simulink model "topology2_module"  (R2013a)
settings: Solver=ode4  StartTime=0.0  StopTime=0.02  FixedStep=Ts  RelTol=1e-3
values from neighbouring files (symbols this model uses):
  enable = zeros(1,max_number_module)    [immd_base_varyingmod.m]
  Lload = Xload/wout_fund    [acemp_sixth.m]    (also in immd_base_varyingmod.m = Xload/wout; immd_design_elen.m = Xload/wout; immd_efficiency.m = Xload/wout; immd_simulation_base.m)
  ma = 1    [IMMD_design_tool_v01.m]    (also in IMMD_design_tool_v02.m = 0.9; immd_base_varyingmod.m; immd_design_elen.m = 0.8; immd_efficiency.m = 0.85)
  phase = zeros(1,max_number_module)    [immd_base_varyingmod.m]    (also in immd_design_elen.m = [0 0 0 0]; immd_simulation_base.m = zeros(1,n))
  Rload = Zload*pf    [acemp_sixth.m]    (also in immd_base_varyingmod.m; immd_design_elen.m; immd_efficiency.m; immd_simulation_base.m)
  Ts = 1e-6    (= 1e-06)    [acemp_sixth.m]    (also in immd_base_varyingmod.m = 1e-05; immd_design_elen.m; immd_efficiency.m; immd_simulation_base.m)
  Vdc = (3/pi)*Vs_ll*sqrt(2)    [IMMD_design_tool_v01.m]    (also in IMMD_design_tool_v02.m; acemp_sixth.m = 400; immd_base_varyingmod.m = 400; immd_capacitor_rms_current.m = 400)
  wout = 2*pi*fout    (= 314.159265359)    [immd_base_varyingmod.m]    (also in immd_design_elen.m; immd_efficiency.m; immd_simulation_base.m)
libraries: powerlib x76, powerlib_meascontrol x26
settings Model: Creator=ugurm  LastModifiedBy=ugurm

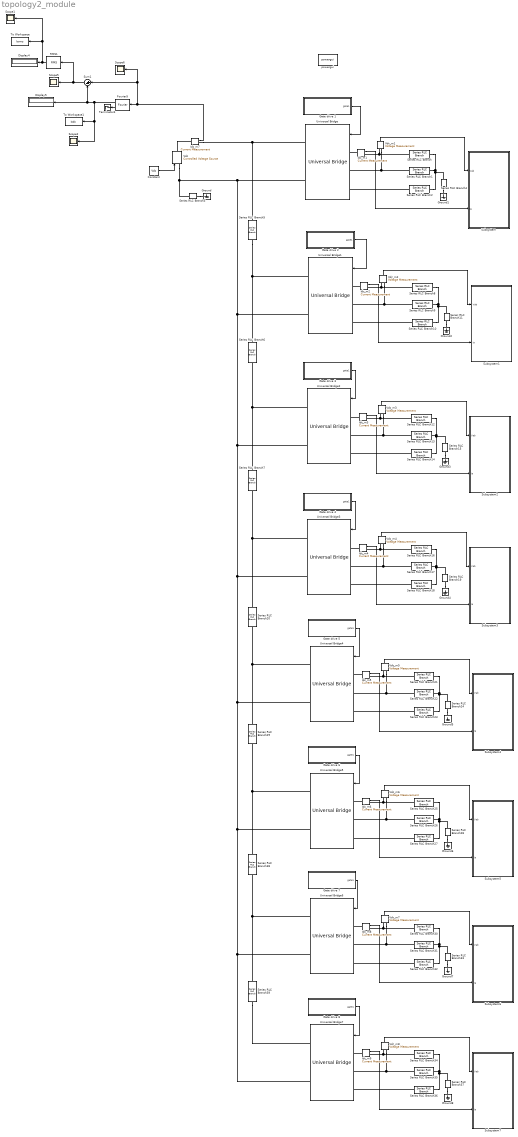
== system topology2_module ==
  Constant : Constant  Value=Vdc
  Display4 : Display
  Display5 : Display
  Fourier5 : powerlib_meascontrol/Measurements/Fourier  Freq=fout  n=0  InInit=[20, 0]  Ts=Ts
  Gate drive 1 : Subsystem
  Gate drive 2 : Subsystem
  Gate drive 3 : Subsystem
  Gate drive 4 : Subsystem
  Gate drive 5 : Subsystem
  Gate drive 6 : Subsystem
  Gate drive 7 : Subsystem
  Gate drive 8 : Subsystem
  Ground{,1..8} (9 alike) : powerlib/Elements/Ground  LConnTagsString=a
  Idc_m{1..9} (9 alike) : powerlib/Measurements/Current Measurement  PhasorSimulation=off  OutputType=Complex  PSBequivalent=0
  RMS1 : powerlib_meascontrol/Measurements/RMS  TrueRMS=on  Freq=50  RMSInit=25  Ts=Ts
  Scope{1..2,5..6} (4 alike) : Scope
      Scope1 settings: YMin=8.8  YMax=10.2
      Scope2 settings: YMin=-25  YMax=40  SaveName=ScopeData3
      Scope5 settings: YMin=-40  YMax=40
      Scope6 settings: YMin=-35  YMax=60  SaveName=ScopeData2
  Series RLC Branch{,1..2,8..10,12..14,16..18,21..23,25..27,30..32,34..36} (24 alike) : powerlib/Elements/Series RLC Branch  LConnTagsString=__new0  RConnTagsString=__new0  BranchType=RL  Resistance=Rload  Inductance=Lload  SetiL0=off  InitialCurrent=0  Capacitance=1e-6  Setx0=off  InitialVoltage=0  Measurements=None
  Series RLC Branch{3..4,11,15,19,24,28,33,37} (9 alike) : powerlib/Elements/Series RLC Branch  LConnTagsString=__new0  RConnTagsString=__new0  BranchType=R  Resistance=1e12  Inductance=Lload  SetiL0=off  InitialCurrent=0  Capacitance=1e-6  Setx0=off  InitialVoltage=0  Measurements=None
  Series RLC Branch{5..7,20,29,38..39} (7 alike) : powerlib/Elements/Series RLC Branch  LConnTagsString=__new0  RConnTagsString=__new0  BranchType=RL  Resistance=1e-6  Inductance=1e-9  SetiL0=off  InitialCurrent=0  Capacitance=1e-6  Setx0=off  InitialVoltage=0  Measurements=None
  Subsystem : Subsystem
  Subsystem1 : Subsystem
  Subsystem2 : Subsystem
  Subsystem3 : Subsystem
  Subsystem4 : Subsystem
  Subsystem5 : Subsystem
  Subsystem6 : Subsystem
  Subsystem7 : Subsystem
  Sum1 : Sum  Inputs=|+-
  Terminator4 : Terminator
  To Workspace : ToWorkspace  VariableName=Icrms  SampleTime=-1
  To Workspace1 : ToWorkspace  VariableName=Icdc  SampleTime=-1
  Universal Bridge{,1..7} (8 alike) : powerlib/Power Electronics/Universal Bridge  Arms=3  SnubberResistance=1e5  SnubberCapacitance=inf  Device=IGBT / Diodes  Ron=1e-6  Lon=0  ForwardVoltages="[  0  0  ]"  ForwardVoltage=0  GTOparameters=[ 10e-6 , 20e-6 ]  IGBTparameters=[0,0]  Measurements=None  Measurements_2=None  converterType=Rectifier
  Vdc : powerlib/Electrical Sources/Controlled Voltage Source  Initialize=off  Source_Type=DC  Amplitude=200  Phase=0  Frequency=0  Measurements=None
  Vdc_m{1..8} (8 alike) : powerlib/Measurements/Voltage Measurement  PhasorSimulation=off  OutputType=Complex  PSBequivalent=0
  powergui : powerlib/powergui  Priority=1  SimulationMode=Discrete  SolverType=Tustin  SampleTime=Ts  frequency=60  SPID=off  DisableSnubberDevices=off  DisableRonSwitches=off  DisableVfSwitches=off  SwTol=0  Interpol=off  DisplayEquations=off  frequencyindice=0  Pbase=100e6  ErrMax=1e-4  Iterations=50  UnitsV=kV  UnitsW=MW  FunctionMessages=off  echomessages=off  HookPort=off  EnableUseOfTLC=off  x0status=blocks  RestoreLinks=warning  ResistiveCurrentMeasurement=off  Frange=[0:2:500]  Ylog=off  Xlog=on  ShowGrid=off  save=off  variable=ZData  structure=ScopeData17  ZoomFFT=off  StartTime=0.1  cycles=50  DisplayStyle=1  fundamental=1000  FreqAxis=off  MaxFrequency=10000  frequencyindicesteady=1  RmsSteady=1  display=off  Ts=0  methode=off
  wires:
  Gate drive 1/1(gate1) -> Universal Bridge/1
  Vdc_m1/1 -> Subsystem/1(Vab)
  Idc_m1/1 -> Subsystem/2(Ia)
  Constant/1 -> Vdc/1
  Idc_m7/1 -> Scope6/1, Sum1/1, Fourier5/1
  Fourier5/2 -> Terminator4/1
  RMS1/1 -> Scope1/1, To Workspace/1, Display4/1
  Fourier5/1 -> Scope2/1, To Workspace1/1, Sum1/2, Display5/1
  Sum1/1 -> RMS1/1, Scope5/1
  Gate drive 2/1(gate1) -> Universal Bridge1/1
  Vdc_m2/1 -> Subsystem1/1(Vab)
  Idc_m2/1 -> Subsystem1/2(Ia)
  Gate drive 3/1(gate1) -> Universal Bridge2/1
  Vdc_m3/1 -> Subsystem2/1(Vab)
  Idc_m3/1 -> Subsystem2/2(Ia)
  Gate drive 4/1(gate1) -> Universal Bridge3/1
  Vdc_m4/1 -> Subsystem3/1(Vab)
  Idc_m4/1 -> Subsystem3/2(Ia)
  Gate drive 5/1(gate1) -> Universal Bridge4/1
  Vdc_m5/1 -> Subsystem4/1(Vab)
  Idc_m5/1 -> Subsystem4/2(Ia)
  Gate drive 6/1(gate1) -> Universal Bridge5/1
  Vdc_m6/1 -> Subsystem5/1(Vab)
  Idc_m6/1 -> Subsystem5/2(Ia)
  Gate drive 7/1(gate1) -> Universal Bridge6/1
  Vdc_m7/1 -> Subsystem6/1(Vab)
  Idc_m8/1 -> Subsystem6/2(Ia)
  Gate drive 8/1(gate1) -> Universal Bridge7/1
  Vdc_m8/1 -> Subsystem7/1(Vab)
  Idc_m9/1 -> Subsystem7/2(Ia)
  connections:
  Idc_m7/RConn1 -- Series RLC Branch5/LConn1 -- Universal Bridge/RConn1
  Idc_m1/LConn1 -- Universal Bridge/LConn1
  Series RLC Branch1/LConn1 -- Universal Bridge/LConn2 -- Vdc_m1/LConn2
  Series RLC Branch2/LConn1 -- Universal Bridge/LConn3
  Series RLC Branch/LConn1 -- Idc_m1/RConn1 -- Vdc_m1/LConn1
  Series RLC Branch/RConn1 -- Series RLC Branch4/LConn1 -- Series RLC Branch2/RConn1 -- Series RLC Branch1/RConn1
  Series RLC Branch4/RConn1 -- Ground1/LConn1
  Series RLC Branch5/RConn1 -- Series RLC Branch6/LConn1 -- Universal Bridge1/RConn1
  Universal Bridge2/RConn1 -- Series RLC Branch6/RConn1 -- Series RLC Branch7/LConn1
  Idc_m7/LConn1 -- Vdc/RConn1
  Series RLC Branch3/RConn1 -- Ground/LConn1
  Vdc/LConn1 -- Series RLC Branch3/LConn1 -- Universal Bridge7/RConn2 -- Universal Bridge6/RConn2 -- Universal Bridge5/RConn2 -- Universal Bridge4/RConn2 -- Universal Bridge3/RConn2 -- Universal Bridge2/RConn2 -- Universal Bridge1/RConn2 -- Universal Bridge/RConn2
  Vdc_m2/LConn2 -- Universal Bridge1/LConn2 -- Series RLC Branch9/LConn1
  Vdc_m2/LConn1 -- Series RLC Branch8/LConn1 -- Idc_m2/RConn1
  Series RLC Branch10/RConn1 -- Series RLC Branch8/RConn1 -- Series RLC Branch9/RConn1 -- Series RLC Branch11/LConn1
  Series RLC Branch10/LConn1 -- Universal Bridge1/LConn3
  Idc_m2/LConn1 -- Universal Bridge1/LConn1
  Series RLC Branch11/RConn1 -- Ground2/LConn1
  Vdc_m3/LConn2 -- Universal Bridge2/LConn2 -- Series RLC Branch13/LConn1
  Vdc_m3/LConn1 -- Series RLC Branch12/LConn1 -- Idc_m3/RConn1
  Series RLC Branch14/RConn1 -- Series RLC Branch12/RConn1 -- Series RLC Branch13/RConn1 -- Series RLC Branch15/LConn1
  Series RLC Branch14/LConn1 -- Universal Bridge2/LConn3
  Idc_m3/LConn1 -- Universal Bridge2/LConn1
  Series RLC Branch15/RConn1 -- Ground3/LConn1
  Vdc_m4/LConn2 -- Universal Bridge3/LConn2 -- Series RLC Branch17/LConn1
  Vdc_m4/LConn1 -- Series RLC Branch16/LConn1 -- Idc_m4/RConn1
  Series RLC Branch18/RConn1 -- Series RLC Branch16/RConn1 -- Series RLC Branch17/RConn1 -- Series RLC Branch19/LConn1
  Series RLC Branch18/LConn1 -- Universal Bridge3/LConn3
  Idc_m4/LConn1 -- Universal Bridge3/LConn1
  Series RLC Branch19/RConn1 -- Ground4/LConn1
  Universal Bridge3/RConn1 -- Series RLC Branch20/LConn1 -- Series RLC Branch7/RConn1
  Vdc_m5/LConn2 -- Universal Bridge4/LConn2 -- Series RLC Branch22/LConn1
  Vdc_m5/LConn1 -- Series RLC Branch21/LConn1 -- Idc_m5/RConn1
  Series RLC Branch23/RConn1 -- Series RLC Branch24/LConn1 -- Series RLC Branch21/RConn1 -- Series RLC Branch22/RConn1
  Series RLC Branch23/LConn1 -- Universal Bridge4/LConn3
  Idc_m5/LConn1 -- Universal Bridge4/LConn1
  Series RLC Branch24/RConn1 -- Ground5/LConn1
  Universal Bridge4/RConn1 -- Series RLC Branch20/RConn1 -- Series RLC Branch29/LConn1
  Vdc_m6/LConn2 -- Universal Bridge5/LConn2 -- Series RLC Branch26/LConn1
  Vdc_m6/LConn1 -- Series RLC Branch25/LConn1 -- Idc_m6/RConn1
  Series RLC Branch26/RConn1 -- Series RLC Branch25/RConn1 -- Series RLC Branch28/LConn1 -- Series RLC Branch27/RConn1
  Idc_m6/LConn1 -- Universal Bridge5/LConn1
  Series RLC Branch27/LConn1 -- Universal Bridge5/LConn3
  Series RLC Branch28/RConn1 -- Ground6/LConn1
  Universal Bridge5/RConn1 -- Series RLC Branch29/RConn1 -- Series RLC Branch38/LConn1
  Vdc_m7/LConn2 -- Universal Bridge6/LConn2 -- Series RLC Branch31/LConn1
  Vdc_m7/LConn1 -- Series RLC Branch30/LConn1 -- Idc_m8/RConn1
  Series RLC Branch31/RConn1 -- Series RLC Branch30/RConn1 -- Series RLC Branch33/LConn1 -- Series RLC Branch32/RConn1
  Vdc_m8/LConn2 -- Universal Bridge7/LConn2 -- Series RLC Branch35/LConn1
  Vdc_m8/LConn1 -- Series RLC Branch34/LConn1 -- Idc_m9/RConn1
  Series RLC Branch36/RConn1 -- Series RLC Branch37/LConn1 -- Series RLC Branch34/RConn1 -- Series RLC Branch35/RConn1
  Series RLC Branch33/RConn1 -- Ground7/LConn1
  Series RLC Branch37/RConn1 -- Ground8/LConn1
  Series RLC Branch36/LConn1 -- Universal Bridge7/LConn3
  Idc_m9/LConn1 -- Universal Bridge7/LConn1
  Idc_m8/LConn1 -- Universal Bridge6/LConn1
  Series RLC Branch39/RConn1 -- Universal Bridge7/RConn1
  Series RLC Branch32/LConn1 -- Universal Bridge6/LConn3
  Universal Bridge6/RConn1 -- Series RLC Branch38/RConn1 -- Series RLC Branch39/LConn1

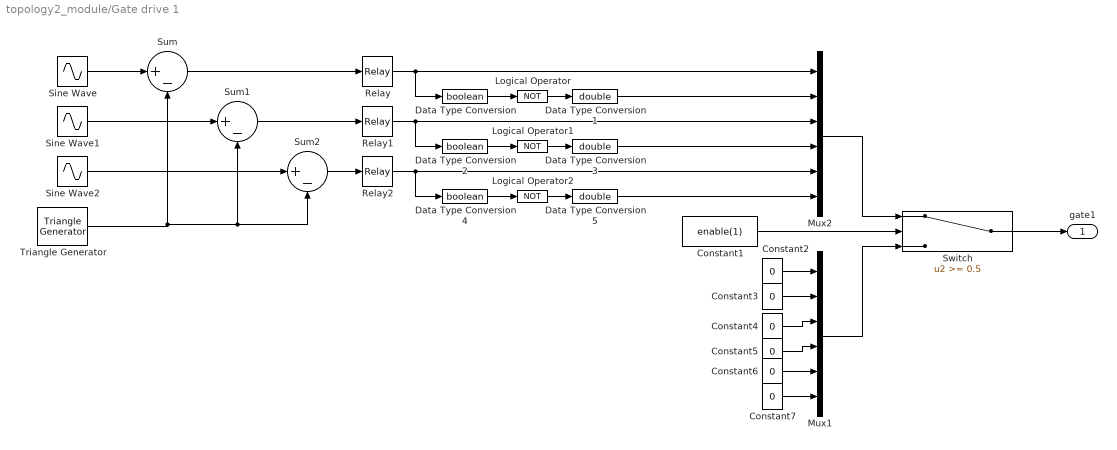
== system topology2_module/Gate drive 1 ==
  Constant1 : Constant  Value=enable(1)
  Constant{2..7} (6 alike) : Constant  Value=0
  Data Type Conversion : DataTypeConversion  OutDataTypeStr=boolean
  Data Type Conversion1 : DataTypeConversion  OutDataTypeStr=double
  Data Type Conversion2 : DataTypeConversion  OutDataTypeStr=boolean
  Data Type Conversion3 : DataTypeConversion  OutDataTypeStr=double
  Data Type Conversion4 : DataTypeConversion  OutDataTypeStr=boolean
  Data Type Conversion5 : DataTypeConversion  OutDataTypeStr=double
  Logical Operator : Logic  Operator=NOT  AllPortsSameDT=off  OutDataTypeStr=boolean
  Logical Operator1 : Logic  Operator=NOT  AllPortsSameDT=off  OutDataTypeStr=boolean
  Logical Operator2 : Logic  Operator=NOT  AllPortsSameDT=off  OutDataTypeStr=boolean
  Mux1 : Mux  Inputs=6
  Mux2 : Mux  Inputs=6
  Relay : Relay
  Relay1 : Relay
  Relay2 : Relay
  Sine Wave : Sin  Amplitude=ma  Frequency=wout  SampleTime=0
  Sine Wave1 : Sin  Amplitude=ma  Frequency=wout  Phase=-2*pi/3  SampleTime=0
  Sine Wave2 : Sin  Amplitude=ma  Frequency=wout  Phase=2*pi/3  SampleTime=0
  Sum : Sum  Inputs=|+-
  Sum1 : Sum  Inputs=|+-
  Sum2 : Sum  Inputs=|+-
  Switch : Switch  Threshold=0.5
  Triangle Generator : powerlib_meascontrol/Pulse & Signal Generators/Triangle Generator  Freq=fsw  Phase=phase(1)  Ts=Ts
  gate1 : Outport
  wires:
  Sine Wave/1 -> Sum/1
  Triangle Generator/1 -> Sum1/2, Sum2/2, Sum/2
  Sine Wave1/1 -> Sum1/1
  Sine Wave2/1 -> Sum2/1
  Sum/1 -> Relay/1
  Sum1/1 -> Relay1/1
  Sum2/1 -> Relay2/1
  Data Type Conversion/1 -> Logical Operator/1
  Relay/1 -> Data Type Conversion/1, Mux2/1
  Logical Operator/1 -> Data Type Conversion1/1
  Data Type Conversion1/1 -> Mux2/2
  Data Type Conversion2/1 -> Logical Operator1/1
  Relay1/1 -> Data Type Conversion2/1, Mux2/3
  Logical Operator1/1 -> Data Type Conversion3/1
  Data Type Conversion3/1 -> Mux2/4
  Data Type Conversion4/1 -> Logical Operator2/1
  Relay2/1 -> Data Type Conversion4/1, Mux2/5
  Logical Operator2/1 -> Data Type Conversion5/1
  Data Type Conversion5/1 -> Mux2/6
  Constant1/1 -> Switch/2
  Constant2/1 -> Mux1/1
  Constant3/1 -> Mux1/2
  Constant4/1 -> Mux1/3
  Constant5/1 -> Mux1/4
  Constant7/1 -> Mux1/6
  Constant6/1 -> Mux1/5
  Mux1/1 -> Switch/3
  Mux2/1 -> Switch/1
  Switch/1 -> gate1/1

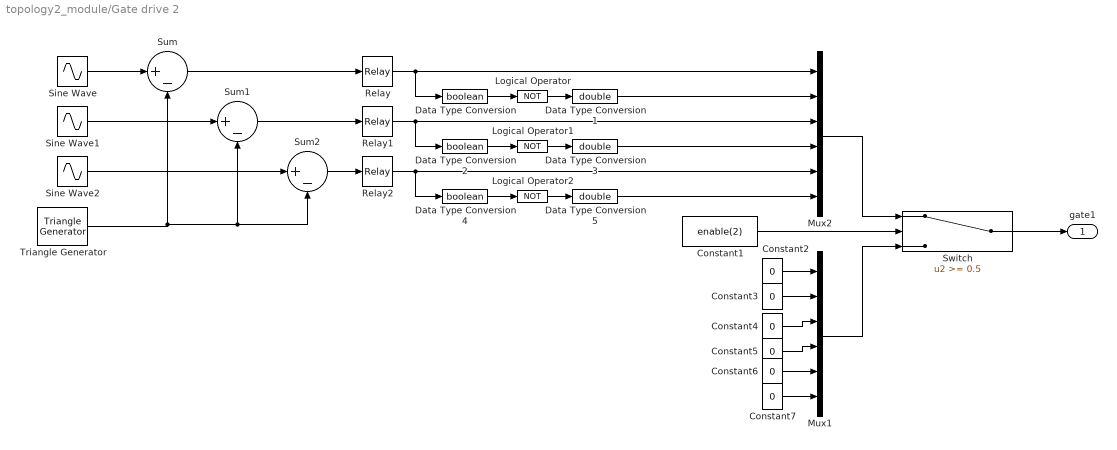
== system topology2_module/Gate drive 2 ==
  Constant1 : Constant  Value=enable(2)
  Constant{2..7} (6 alike) : Constant  Value=0
  Data Type Conversion : DataTypeConversion  OutDataTypeStr=boolean
  Data Type Conversion1 : DataTypeConversion  OutDataTypeStr=double
  Data Type Conversion2 : DataTypeConversion  OutDataTypeStr=boolean
  Data Type Conversion3 : DataTypeConversion  OutDataTypeStr=double
  Data Type Conversion4 : DataTypeConversion  OutDataTypeStr=boolean
  Data Type Conversion5 : DataTypeConversion  OutDataTypeStr=double
  Logical Operator : Logic  Operator=NOT  AllPortsSameDT=off  OutDataTypeStr=boolean
  Logical Operator1 : Logic  Operator=NOT  AllPortsSameDT=off  OutDataTypeStr=boolean
  Logical Operator2 : Logic  Operator=NOT  AllPortsSameDT=off  OutDataTypeStr=boolean
  Mux1 : Mux  Inputs=6
  Mux2 : Mux  Inputs=6
  Relay : Relay
  Relay1 : Relay
  Relay2 : Relay
  Sine Wave : Sin  Amplitude=ma  Frequency=wout  SampleTime=0
  Sine Wave1 : Sin  Amplitude=ma  Frequency=wout  Phase=-2*pi/3  SampleTime=0
  Sine Wave2 : Sin  Amplitude=ma  Frequency=wout  Phase=2*pi/3  SampleTime=0
  Sum : Sum  Inputs=|+-
  Sum1 : Sum  Inputs=|+-
  Sum2 : Sum  Inputs=|+-
  Switch : Switch  Threshold=0.5
  Triangle Generator : powerlib_meascontrol/Pulse & Signal Generators/Triangle Generator  Freq=fsw  Phase=phase(2)  Ts=Ts
  gate1 : Outport
  wires:
  Sine Wave/1 -> Sum/1
  Triangle Generator/1 -> Sum1/2, Sum2/2, Sum/2
  Sine Wave1/1 -> Sum1/1
  Sine Wave2/1 -> Sum2/1
  Sum/1 -> Relay/1
  Sum1/1 -> Relay1/1
  Sum2/1 -> Relay2/1
  Data Type Conversion/1 -> Logical Operator/1
  Relay/1 -> Data Type Conversion/1, Mux2/1
  Logical Operator/1 -> Data Type Conversion1/1
  Data Type Conversion1/1 -> Mux2/2
  Data Type Conversion2/1 -> Logical Operator1/1
  Relay1/1 -> Data Type Conversion2/1, Mux2/3
  Logical Operator1/1 -> Data Type Conversion3/1
  Data Type Conversion3/1 -> Mux2/4
  Data Type Conversion4/1 -> Logical Operator2/1
  Relay2/1 -> Data Type Conversion4/1, Mux2/5
  Logical Operator2/1 -> Data Type Conversion5/1
  Data Type Conversion5/1 -> Mux2/6
  Constant1/1 -> Switch/2
  Constant2/1 -> Mux1/1
  Constant3/1 -> Mux1/2
  Constant4/1 -> Mux1/3
  Constant5/1 -> Mux1/4
  Constant7/1 -> Mux1/6
  Constant6/1 -> Mux1/5
  Mux1/1 -> Switch/3
  Mux2/1 -> Switch/1
  Switch/1 -> gate1/1

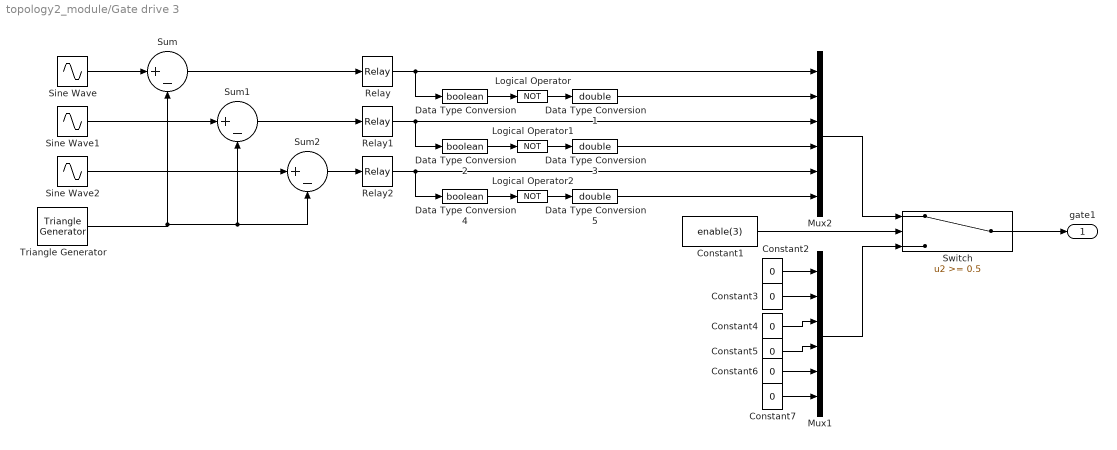
== system topology2_module/Gate drive 3 ==
  Constant1 : Constant  Value=enable(3)
  Constant{2..7} (6 alike) : Constant  Value=0
  Data Type Conversion : DataTypeConversion  OutDataTypeStr=boolean
  Data Type Conversion1 : DataTypeConversion  OutDataTypeStr=double
  Data Type Conversion2 : DataTypeConversion  OutDataTypeStr=boolean
  Data Type Conversion3 : DataTypeConversion  OutDataTypeStr=double
  Data Type Conversion4 : DataTypeConversion  OutDataTypeStr=boolean
  Data Type Conversion5 : DataTypeConversion  OutDataTypeStr=double
  Logical Operator : Logic  Operator=NOT  AllPortsSameDT=off  OutDataTypeStr=boolean
  Logical Operator1 : Logic  Operator=NOT  AllPortsSameDT=off  OutDataTypeStr=boolean
  Logical Operator2 : Logic  Operator=NOT  AllPortsSameDT=off  OutDataTypeStr=boolean
  Mux1 : Mux  Inputs=6
  Mux2 : Mux  Inputs=6
  Relay : Relay
  Relay1 : Relay
  Relay2 : Relay
  Sine Wave : Sin  Amplitude=ma  Frequency=wout  SampleTime=0
  Sine Wave1 : Sin  Amplitude=ma  Frequency=wout  Phase=-2*pi/3  SampleTime=0
  Sine Wave2 : Sin  Amplitude=ma  Frequency=wout  Phase=2*pi/3  SampleTime=0
  Sum : Sum  Inputs=|+-
  Sum1 : Sum  Inputs=|+-
  Sum2 : Sum  Inputs=|+-
  Switch : Switch  Threshold=0.5
  Triangle Generator : powerlib_meascontrol/Pulse & Signal Generators/Triangle Generator  Freq=fsw  Phase=phase(3)  Ts=Ts
  gate1 : Outport
  wires:
  Sine Wave/1 -> Sum/1
  Triangle Generator/1 -> Sum1/2, Sum2/2, Sum/2
  Sine Wave1/1 -> Sum1/1
  Sine Wave2/1 -> Sum2/1
  Sum/1 -> Relay/1
  Sum1/1 -> Relay1/1
  Sum2/1 -> Relay2/1
  Data Type Conversion/1 -> Logical Operator/1
  Relay/1 -> Data Type Conversion/1, Mux2/1
  Logical Operator/1 -> Data Type Conversion1/1
  Data Type Conversion1/1 -> Mux2/2
  Data Type Conversion2/1 -> Logical Operator1/1
  Relay1/1 -> Data Type Conversion2/1, Mux2/3
  Logical Operator1/1 -> Data Type Conversion3/1
  Data Type Conversion3/1 -> Mux2/4
  Data Type Conversion4/1 -> Logical Operator2/1
  Relay2/1 -> Data Type Conversion4/1, Mux2/5
  Logical Operator2/1 -> Data Type Conversion5/1
  Data Type Conversion5/1 -> Mux2/6
  Constant1/1 -> Switch/2
  Constant2/1 -> Mux1/1
  Constant3/1 -> Mux1/2
  Constant4/1 -> Mux1/3
  Constant5/1 -> Mux1/4
  Constant7/1 -> Mux1/6
  Constant6/1 -> Mux1/5
  Mux1/1 -> Switch/3
  Mux2/1 -> Switch/1
  Switch/1 -> gate1/1

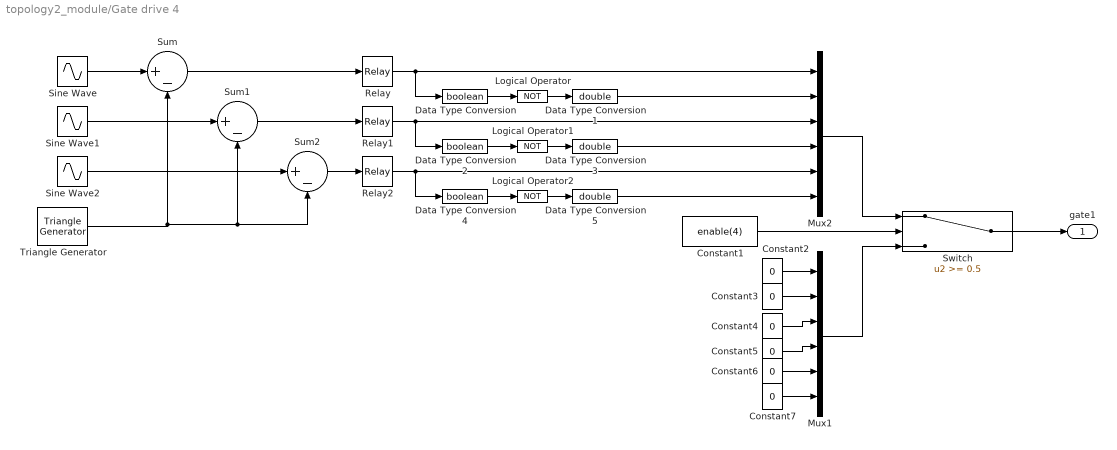
== system topology2_module/Gate drive 4 ==
  Constant1 : Constant  Value=enable(4)
  Constant{2..7} (6 alike) : Constant  Value=0
  Data Type Conversion : DataTypeConversion  OutDataTypeStr=boolean
  Data Type Conversion1 : DataTypeConversion  OutDataTypeStr=double
  Data Type Conversion2 : DataTypeConversion  OutDataTypeStr=boolean
  Data Type Conversion3 : DataTypeConversion  OutDataTypeStr=double
  Data Type Conversion4 : DataTypeConversion  OutDataTypeStr=boolean
  Data Type Conversion5 : DataTypeConversion  OutDataTypeStr=double
  Logical Operator : Logic  Operator=NOT  AllPortsSameDT=off  OutDataTypeStr=boolean
  Logical Operator1 : Logic  Operator=NOT  AllPortsSameDT=off  OutDataTypeStr=boolean
  Logical Operator2 : Logic  Operator=NOT  AllPortsSameDT=off  OutDataTypeStr=boolean
  Mux1 : Mux  Inputs=6
  Mux2 : Mux  Inputs=6
  Relay : Relay
  Relay1 : Relay
  Relay2 : Relay
  Sine Wave : Sin  Amplitude=ma  Frequency=wout  SampleTime=0
  Sine Wave1 : Sin  Amplitude=ma  Frequency=wout  Phase=-2*pi/3  SampleTime=0
  Sine Wave2 : Sin  Amplitude=ma  Frequency=wout  Phase=2*pi/3  SampleTime=0
  Sum : Sum  Inputs=|+-
  Sum1 : Sum  Inputs=|+-
  Sum2 : Sum  Inputs=|+-
  Switch : Switch  Threshold=0.5
  Triangle Generator : powerlib_meascontrol/Pulse & Signal Generators/Triangle Generator  Freq=fsw  Phase=phase(4)  Ts=Ts
  gate1 : Outport
  wires:
  Sine Wave/1 -> Sum/1
  Triangle Generator/1 -> Sum1/2, Sum2/2, Sum/2
  Sine Wave1/1 -> Sum1/1
  Sine Wave2/1 -> Sum2/1
  Sum/1 -> Relay/1
  Sum1/1 -> Relay1/1
  Sum2/1 -> Relay2/1
  Data Type Conversion/1 -> Logical Operator/1
  Relay/1 -> Data Type Conversion/1, Mux2/1
  Logical Operator/1 -> Data Type Conversion1/1
  Data Type Conversion1/1 -> Mux2/2
  Data Type Conversion2/1 -> Logical Operator1/1
  Relay1/1 -> Data Type Conversion2/1, Mux2/3
  Logical Operator1/1 -> Data Type Conversion3/1
  Data Type Conversion3/1 -> Mux2/4
  Data Type Conversion4/1 -> Logical Operator2/1
  Relay2/1 -> Data Type Conversion4/1, Mux2/5
  Logical Operator2/1 -> Data Type Conversion5/1
  Data Type Conversion5/1 -> Mux2/6
  Constant1/1 -> Switch/2
  Constant2/1 -> Mux1/1
  Constant3/1 -> Mux1/2
  Constant4/1 -> Mux1/3
  Constant5/1 -> Mux1/4
  Constant7/1 -> Mux1/6
  Constant6/1 -> Mux1/5
  Mux1/1 -> Switch/3
  Mux2/1 -> Switch/1
  Switch/1 -> gate1/1

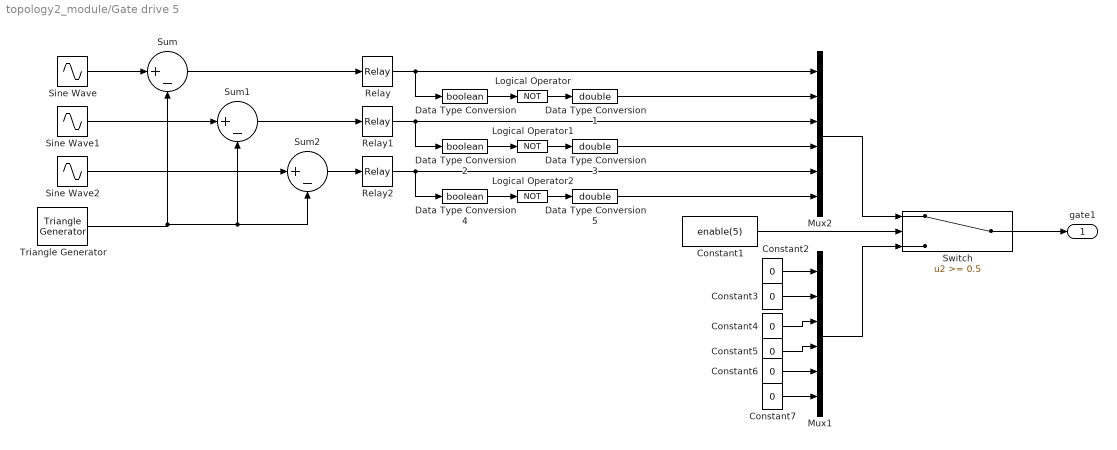
== system topology2_module/Gate drive 5 ==
  Constant1 : Constant  Value=enable(5)
  Constant{2..7} (6 alike) : Constant  Value=0
  Data Type Conversion : DataTypeConversion  OutDataTypeStr=boolean
  Data Type Conversion1 : DataTypeConversion  OutDataTypeStr=double
  Data Type Conversion2 : DataTypeConversion  OutDataTypeStr=boolean
  Data Type Conversion3 : DataTypeConversion  OutDataTypeStr=double
  Data Type Conversion4 : DataTypeConversion  OutDataTypeStr=boolean
  Data Type Conversion5 : DataTypeConversion  OutDataTypeStr=double
  Logical Operator : Logic  Operator=NOT  AllPortsSameDT=off  OutDataTypeStr=boolean
  Logical Operator1 : Logic  Operator=NOT  AllPortsSameDT=off  OutDataTypeStr=boolean
  Logical Operator2 : Logic  Operator=NOT  AllPortsSameDT=off  OutDataTypeStr=boolean
  Mux1 : Mux  Inputs=6
  Mux2 : Mux  Inputs=6
  Relay : Relay
  Relay1 : Relay
  Relay2 : Relay
  Sine Wave : Sin  Amplitude=ma  Frequency=wout  SampleTime=0
  Sine Wave1 : Sin  Amplitude=ma  Frequency=wout  Phase=-2*pi/3  SampleTime=0
  Sine Wave2 : Sin  Amplitude=ma  Frequency=wout  Phase=2*pi/3  SampleTime=0
  Sum : Sum  Inputs=|+-
  Sum1 : Sum  Inputs=|+-
  Sum2 : Sum  Inputs=|+-
  Switch : Switch  Threshold=0.5
  Triangle Generator : powerlib_meascontrol/Pulse & Signal Generators/Triangle Generator  Freq=fsw  Phase=phase(5)  Ts=Ts
  gate1 : Outport
  wires:
  Sine Wave/1 -> Sum/1
  Triangle Generator/1 -> Sum1/2, Sum2/2, Sum/2
  Sine Wave1/1 -> Sum1/1
  Sine Wave2/1 -> Sum2/1
  Sum/1 -> Relay/1
  Sum1/1 -> Relay1/1
  Sum2/1 -> Relay2/1
  Data Type Conversion/1 -> Logical Operator/1
  Relay/1 -> Data Type Conversion/1, Mux2/1
  Logical Operator/1 -> Data Type Conversion1/1
  Data Type Conversion1/1 -> Mux2/2
  Data Type Conversion2/1 -> Logical Operator1/1
  Relay1/1 -> Data Type Conversion2/1, Mux2/3
  Logical Operator1/1 -> Data Type Conversion3/1
  Data Type Conversion3/1 -> Mux2/4
  Data Type Conversion4/1 -> Logical Operator2/1
  Relay2/1 -> Data Type Conversion4/1, Mux2/5
  Logical Operator2/1 -> Data Type Conversion5/1
  Data Type Conversion5/1 -> Mux2/6
  Constant1/1 -> Switch/2
  Constant2/1 -> Mux1/1
  Constant3/1 -> Mux1/2
  Constant4/1 -> Mux1/3
  Constant5/1 -> Mux1/4
  Constant7/1 -> Mux1/6
  Constant6/1 -> Mux1/5
  Mux1/1 -> Switch/3
  Mux2/1 -> Switch/1
  Switch/1 -> gate1/1

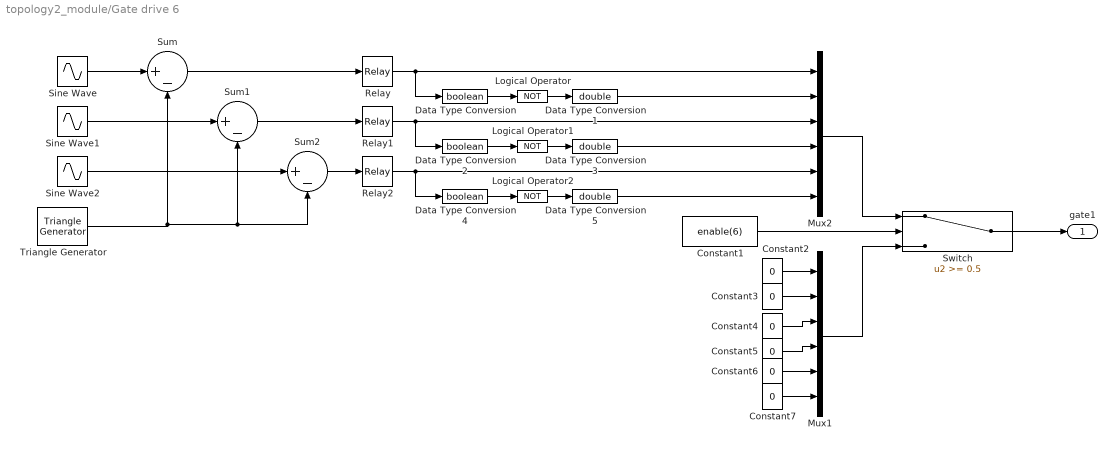
== system topology2_module/Gate drive 6 ==
  Constant1 : Constant  Value=enable(6)
  Constant{2..7} (6 alike) : Constant  Value=0
  Data Type Conversion : DataTypeConversion  OutDataTypeStr=boolean
  Data Type Conversion1 : DataTypeConversion  OutDataTypeStr=double
  Data Type Conversion2 : DataTypeConversion  OutDataTypeStr=boolean
  Data Type Conversion3 : DataTypeConversion  OutDataTypeStr=double
  Data Type Conversion4 : DataTypeConversion  OutDataTypeStr=boolean
  Data Type Conversion5 : DataTypeConversion  OutDataTypeStr=double
  Logical Operator : Logic  Operator=NOT  AllPortsSameDT=off  OutDataTypeStr=boolean
  Logical Operator1 : Logic  Operator=NOT  AllPortsSameDT=off  OutDataTypeStr=boolean
  Logical Operator2 : Logic  Operator=NOT  AllPortsSameDT=off  OutDataTypeStr=boolean
  Mux1 : Mux  Inputs=6
  Mux2 : Mux  Inputs=6
  Relay : Relay
  Relay1 : Relay
  Relay2 : Relay
  Sine Wave : Sin  Amplitude=ma  Frequency=wout  SampleTime=0
  Sine Wave1 : Sin  Amplitude=ma  Frequency=wout  Phase=-2*pi/3  SampleTime=0
  Sine Wave2 : Sin  Amplitude=ma  Frequency=wout  Phase=2*pi/3  SampleTime=0
  Sum : Sum  Inputs=|+-
  Sum1 : Sum  Inputs=|+-
  Sum2 : Sum  Inputs=|+-
  Switch : Switch  Threshold=0.5
  Triangle Generator : powerlib_meascontrol/Pulse & Signal Generators/Triangle Generator  Freq=fsw  Phase=phase(6)  Ts=Ts
  gate1 : Outport
  wires:
  Sine Wave/1 -> Sum/1
  Triangle Generator/1 -> Sum1/2, Sum2/2, Sum/2
  Sine Wave1/1 -> Sum1/1
  Sine Wave2/1 -> Sum2/1
  Sum/1 -> Relay/1
  Sum1/1 -> Relay1/1
  Sum2/1 -> Relay2/1
  Data Type Conversion/1 -> Logical Operator/1
  Relay/1 -> Data Type Conversion/1, Mux2/1
  Logical Operator/1 -> Data Type Conversion1/1
  Data Type Conversion1/1 -> Mux2/2
  Data Type Conversion2/1 -> Logical Operator1/1
  Relay1/1 -> Data Type Conversion2/1, Mux2/3
  Logical Operator1/1 -> Data Type Conversion3/1
  Data Type Conversion3/1 -> Mux2/4
  Data Type Conversion4/1 -> Logical Operator2/1
  Relay2/1 -> Data Type Conversion4/1, Mux2/5
  Logical Operator2/1 -> Data Type Conversion5/1
  Data Type Conversion5/1 -> Mux2/6
  Constant1/1 -> Switch/2
  Constant2/1 -> Mux1/1
  Constant3/1 -> Mux1/2
  Constant4/1 -> Mux1/3
  Constant5/1 -> Mux1/4
  Constant7/1 -> Mux1/6
  Constant6/1 -> Mux1/5
  Mux1/1 -> Switch/3
  Mux2/1 -> Switch/1
  Switch/1 -> gate1/1

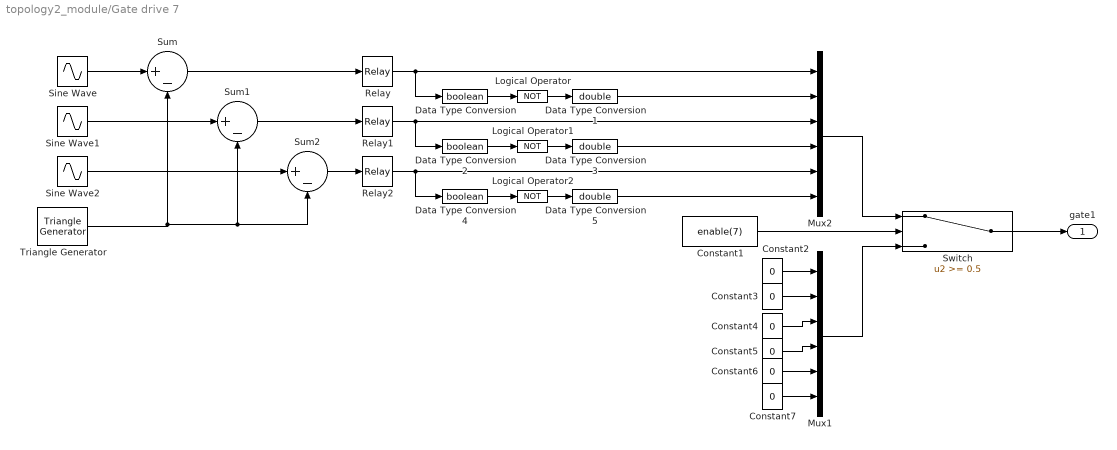
== system topology2_module/Gate drive 7 ==
  Constant1 : Constant  Value=enable(7)
  Constant{2..7} (6 alike) : Constant  Value=0
  Data Type Conversion : DataTypeConversion  OutDataTypeStr=boolean
  Data Type Conversion1 : DataTypeConversion  OutDataTypeStr=double
  Data Type Conversion2 : DataTypeConversion  OutDataTypeStr=boolean
  Data Type Conversion3 : DataTypeConversion  OutDataTypeStr=double
  Data Type Conversion4 : DataTypeConversion  OutDataTypeStr=boolean
  Data Type Conversion5 : DataTypeConversion  OutDataTypeStr=double
  Logical Operator : Logic  Operator=NOT  AllPortsSameDT=off  OutDataTypeStr=boolean
  Logical Operator1 : Logic  Operator=NOT  AllPortsSameDT=off  OutDataTypeStr=boolean
  Logical Operator2 : Logic  Operator=NOT  AllPortsSameDT=off  OutDataTypeStr=boolean
  Mux1 : Mux  Inputs=6
  Mux2 : Mux  Inputs=6
  Relay : Relay
  Relay1 : Relay
  Relay2 : Relay
  Sine Wave : Sin  Amplitude=ma  Frequency=wout  SampleTime=0
  Sine Wave1 : Sin  Amplitude=ma  Frequency=wout  Phase=-2*pi/3  SampleTime=0
  Sine Wave2 : Sin  Amplitude=ma  Frequency=wout  Phase=2*pi/3  SampleTime=0
  Sum : Sum  Inputs=|+-
  Sum1 : Sum  Inputs=|+-
  Sum2 : Sum  Inputs=|+-
  Switch : Switch  Threshold=0.5
  Triangle Generator : powerlib_meascontrol/Pulse & Signal Generators/Triangle Generator  Freq=fsw  Phase=phase(7)  Ts=Ts
  gate1 : Outport
  wires:
  Sine Wave/1 -> Sum/1
  Triangle Generator/1 -> Sum1/2, Sum2/2, Sum/2
  Sine Wave1/1 -> Sum1/1
  Sine Wave2/1 -> Sum2/1
  Sum/1 -> Relay/1
  Sum1/1 -> Relay1/1
  Sum2/1 -> Relay2/1
  Data Type Conversion/1 -> Logical Operator/1
  Relay/1 -> Data Type Conversion/1, Mux2/1
  Logical Operator/1 -> Data Type Conversion1/1
  Data Type Conversion1/1 -> Mux2/2
  Data Type Conversion2/1 -> Logical Operator1/1
  Relay1/1 -> Data Type Conversion2/1, Mux2/3
  Logical Operator1/1 -> Data Type Conversion3/1
  Data Type Conversion3/1 -> Mux2/4
  Data Type Conversion4/1 -> Logical Operator2/1
  Relay2/1 -> Data Type Conversion4/1, Mux2/5
  Logical Operator2/1 -> Data Type Conversion5/1
  Data Type Conversion5/1 -> Mux2/6
  Constant1/1 -> Switch/2
  Constant2/1 -> Mux1/1
  Constant3/1 -> Mux1/2
  Constant4/1 -> Mux1/3
  Constant5/1 -> Mux1/4
  Constant7/1 -> Mux1/6
  Constant6/1 -> Mux1/5
  Mux1/1 -> Switch/3
  Mux2/1 -> Switch/1
  Switch/1 -> gate1/1

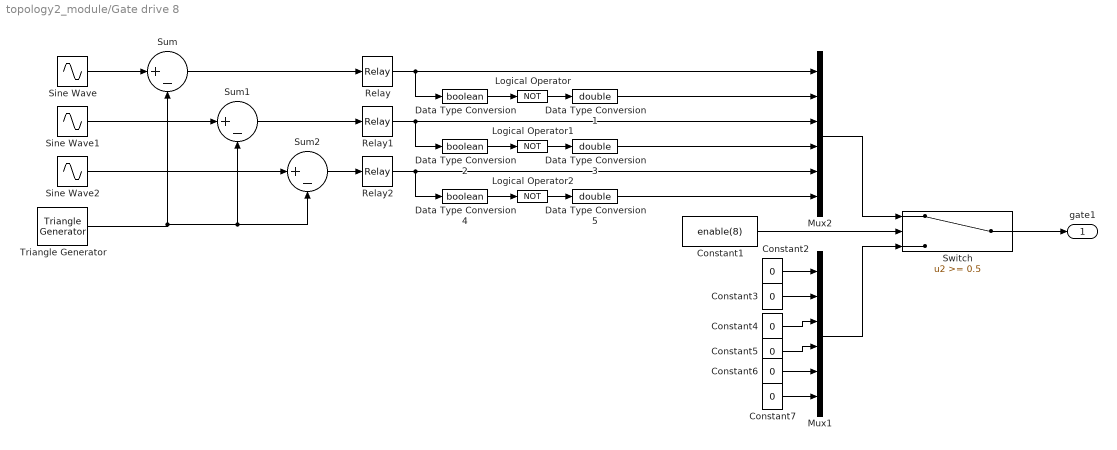
== system topology2_module/Gate drive 8 ==
  Constant1 : Constant  Value=enable(8)
  Constant{2..7} (6 alike) : Constant  Value=0
  Data Type Conversion : DataTypeConversion  OutDataTypeStr=boolean
  Data Type Conversion1 : DataTypeConversion  OutDataTypeStr=double
  Data Type Conversion2 : DataTypeConversion  OutDataTypeStr=boolean
  Data Type Conversion3 : DataTypeConversion  OutDataTypeStr=double
  Data Type Conversion4 : DataTypeConversion  OutDataTypeStr=boolean
  Data Type Conversion5 : DataTypeConversion  OutDataTypeStr=double
  Logical Operator : Logic  Operator=NOT  AllPortsSameDT=off  OutDataTypeStr=boolean
  Logical Operator1 : Logic  Operator=NOT  AllPortsSameDT=off  OutDataTypeStr=boolean
  Logical Operator2 : Logic  Operator=NOT  AllPortsSameDT=off  OutDataTypeStr=boolean
  Mux1 : Mux  Inputs=6
  Mux2 : Mux  Inputs=6
  Relay : Relay
  Relay1 : Relay
  Relay2 : Relay
  Sine Wave : Sin  Amplitude=ma  Frequency=wout  SampleTime=0
  Sine Wave1 : Sin  Amplitude=ma  Frequency=wout  Phase=-2*pi/3  SampleTime=0
  Sine Wave2 : Sin  Amplitude=ma  Frequency=wout  Phase=2*pi/3  SampleTime=0
  Sum : Sum  Inputs=|+-
  Sum1 : Sum  Inputs=|+-
  Sum2 : Sum  Inputs=|+-
  Switch : Switch  Threshold=0.5
  Triangle Generator : powerlib_meascontrol/Pulse & Signal Generators/Triangle Generator  Freq=fsw  Phase=phase(8)  Ts=Ts
  gate1 : Outport
  wires:
  Sine Wave/1 -> Sum/1
  Triangle Generator/1 -> Sum1/2, Sum2/2, Sum/2
  Sine Wave1/1 -> Sum1/1
  Sine Wave2/1 -> Sum2/1
  Sum/1 -> Relay/1
  Sum1/1 -> Relay1/1
  Sum2/1 -> Relay2/1
  Data Type Conversion/1 -> Logical Operator/1
  Relay/1 -> Data Type Conversion/1, Mux2/1
  Logical Operator/1 -> Data Type Conversion1/1
  Data Type Conversion1/1 -> Mux2/2
  Data Type Conversion2/1 -> Logical Operator1/1
  Relay1/1 -> Data Type Conversion2/1, Mux2/3
  Logical Operator1/1 -> Data Type Conversion3/1
  Data Type Conversion3/1 -> Mux2/4
  Data Type Conversion4/1 -> Logical Operator2/1
  Relay2/1 -> Data Type Conversion4/1, Mux2/5
  Logical Operator2/1 -> Data Type Conversion5/1
  Data Type Conversion5/1 -> Mux2/6
  Constant1/1 -> Switch/2
  Constant2/1 -> Mux1/1
  Constant3/1 -> Mux1/2
  Constant4/1 -> Mux1/3
  Constant5/1 -> Mux1/4
  Constant7/1 -> Mux1/6
  Constant6/1 -> Mux1/5
  Mux1/1 -> Switch/3
  Mux2/1 -> Switch/1
  Switch/1 -> gate1/1

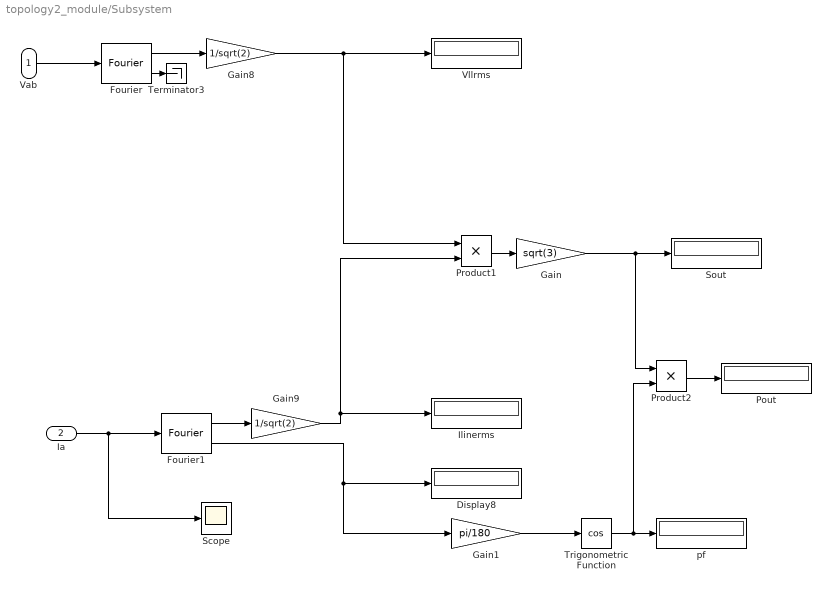
== system topology2_module/Subsystem ==
  Vab : Inport
  Ia : Inport  Port=2
  Display8 : Display
  Fourier : powerlib_meascontrol/Measurements/Fourier  Freq=fout  n=1  InInit=[0, 0]  Ts=Ts
  Fourier1 : powerlib_meascontrol/Measurements/Fourier  Freq=fout  n=1  InInit=[0, 0]  Ts=Ts
  Gain : Gain  Gain=sqrt(3)
  Gain1 : Gain  Gain=pi/180
  Gain8 : Gain  Gain=1/sqrt(2)
  Gain9 : Gain  Gain=1/sqrt(2)
  "Ilinerms " : Display
  Pout : Display
  Product1 : Product
  Product2 : Product
  Scope : Scope
      settings: YMin=-10  YMax=10  SaveName=ScopeData4
  Sout : Display
      settings: Format=short_e
  Terminator3 : Terminator
  Trigonometric Function : Trigonometry  Operator=cos
  "Vllrms " : Display
  pf : Display
  wires:
  Gain8/1 -> Product1/1, "Vllrms "/1
  Gain9/1 -> "Ilinerms "/1, Product1/2
  Ia/1 -> Scope/1, Fourier1/1
  Fourier1/1 -> Gain9/1
  Vab/1 -> Fourier/1
  Fourier/1 -> Gain8/1
  Product1/1 -> Gain/1
  Gain/1 -> Product2/1, Sout/1
  Fourier1/2 -> Gain1/1, Display8/1
  Trigonometric Function/1 -> Product2/2, pf/1
  Gain1/1 -> Trigonometric Function/1
  Product2/1 -> Pout/1
  Fourier/2 -> Terminator3/1

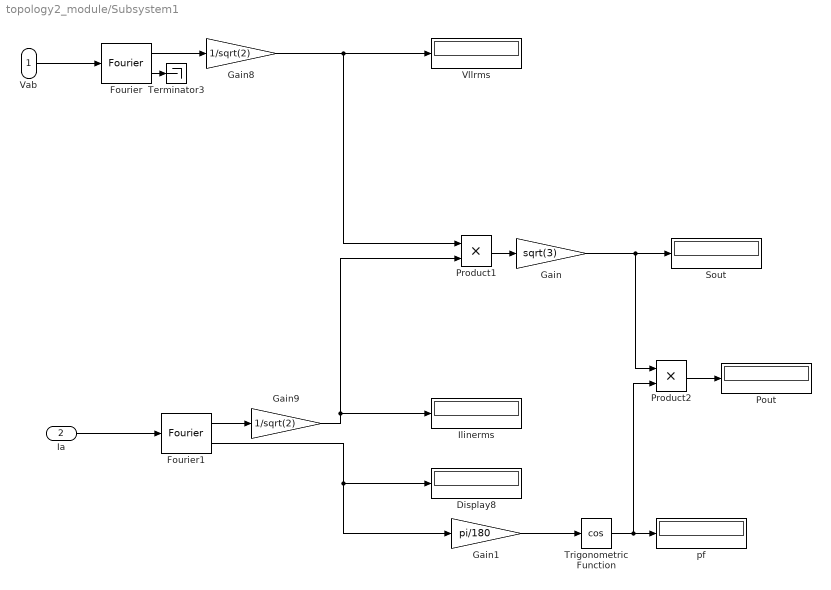
== system topology2_module/Subsystem1 ==
  Vab : Inport
  Ia : Inport  Port=2
  Display8 : Display
  Fourier : powerlib_meascontrol/Measurements/Fourier  Freq=fout  n=1  InInit=[0, 0]  Ts=Ts
  Fourier1 : powerlib_meascontrol/Measurements/Fourier  Freq=fout  n=1  InInit=[0, 0]  Ts=Ts
  Gain : Gain  Gain=sqrt(3)
  Gain1 : Gain  Gain=pi/180
  Gain8 : Gain  Gain=1/sqrt(2)
  Gain9 : Gain  Gain=1/sqrt(2)
  "Ilinerms " : Display
  Pout : Display
  Product1 : Product
  Product2 : Product
  Sout : Display
      settings: Format=short_e
  Terminator3 : Terminator
  Trigonometric Function : Trigonometry  Operator=cos
  "Vllrms " : Display
  pf : Display
  wires:
  Gain8/1 -> Product1/1, "Vllrms "/1
  Gain9/1 -> "Ilinerms "/1, Product1/2
  Ia/1 -> Fourier1/1
  Fourier1/1 -> Gain9/1
  Vab/1 -> Fourier/1
  Fourier/1 -> Gain8/1
  Product1/1 -> Gain/1
  Gain/1 -> Product2/1, Sout/1
  Fourier1/2 -> Gain1/1, Display8/1
  Trigonometric Function/1 -> Product2/2, pf/1
  Gain1/1 -> Trigonometric Function/1
  Product2/1 -> Pout/1
  Fourier/2 -> Terminator3/1

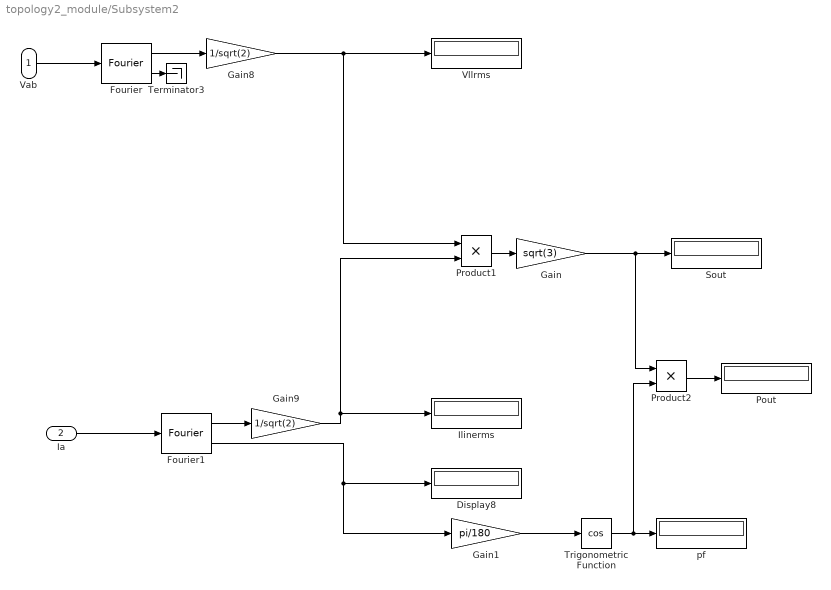
== system topology2_module/Subsystem2 ==
  Vab : Inport
  Ia : Inport  Port=2
  Display8 : Display
  Fourier : powerlib_meascontrol/Measurements/Fourier  Freq=fout  n=1  InInit=[0, 0]  Ts=Ts
  Fourier1 : powerlib_meascontrol/Measurements/Fourier  Freq=fout  n=1  InInit=[0, 0]  Ts=Ts
  Gain : Gain  Gain=sqrt(3)
  Gain1 : Gain  Gain=pi/180
  Gain8 : Gain  Gain=1/sqrt(2)
  Gain9 : Gain  Gain=1/sqrt(2)
  "Ilinerms " : Display
  Pout : Display
  Product1 : Product
  Product2 : Product
  Sout : Display
      settings: Format=short_e
  Terminator3 : Terminator
  Trigonometric Function : Trigonometry  Operator=cos
  "Vllrms " : Display
  pf : Display
  wires:
  Gain8/1 -> Product1/1, "Vllrms "/1
  Gain9/1 -> "Ilinerms "/1, Product1/2
  Ia/1 -> Fourier1/1
  Fourier1/1 -> Gain9/1
  Vab/1 -> Fourier/1
  Fourier/1 -> Gain8/1
  Product1/1 -> Gain/1
  Gain/1 -> Product2/1, Sout/1
  Fourier1/2 -> Gain1/1, Display8/1
  Trigonometric Function/1 -> Product2/2, pf/1
  Gain1/1 -> Trigonometric Function/1
  Product2/1 -> Pout/1
  Fourier/2 -> Terminator3/1

== system topology2_module/Subsystem3 ==
  Vab : Inport
  Ia : Inport  Port=2
  Display8 : Display
  Fourier : powerlib_meascontrol/Measurements/Fourier  Freq=fout  n=1  InInit=[0, 0]  Ts=Ts
  Fourier1 : powerlib_meascontrol/Measurements/Fourier  Freq=fout  n=1  InInit=[0, 0]  Ts=Ts
  Gain : Gain  Gain=sqrt(3)
  Gain1 : Gain  Gain=pi/180
  Gain8 : Gain  Gain=1/sqrt(2)
  Gain9 : Gain  Gain=1/sqrt(2)
  "Ilinerms " : Display
  Pout : Display
  Product1 : Product
  Product2 : Product
  Sout : Display
      settings: Format=short_e
  Terminator3 : Terminator
  Trigonometric Function : Trigonometry  Operator=cos
  "Vllrms " : Display
  pf : Display
  wires:
  Gain8/1 -> Product1/1, "Vllrms "/1
  Gain9/1 -> "Ilinerms "/1, Product1/2
  Ia/1 -> Fourier1/1
  Fourier1/1 -> Gain9/1
  Vab/1 -> Fourier/1
  Fourier/1 -> Gain8/1
  Product1/1 -> Gain/1
  Gain/1 -> Product2/1, Sout/1
  Fourier1/2 -> Gain1/1, Display8/1
  Trigonometric Function/1 -> Product2/2, pf/1
  Gain1/1 -> Trigonometric Function/1
  Product2/1 -> Pout/1
  Fourier/2 -> Terminator3/1

== system topology2_module/Subsystem4 ==
  Vab : Inport
  Ia : Inport  Port=2
  Display8 : Display
  Fourier : powerlib_meascontrol/Measurements/Fourier  Freq=fout  n=1  InInit=[0, 0]  Ts=Ts
  Fourier1 : powerlib_meascontrol/Measurements/Fourier  Freq=fout  n=1  InInit=[0, 0]  Ts=Ts
  Gain : Gain  Gain=sqrt(3)
  Gain1 : Gain  Gain=pi/180
  Gain8 : Gain  Gain=1/sqrt(2)
  Gain9 : Gain  Gain=1/sqrt(2)
  "Ilinerms " : Display
  Pout : Display
  Product1 : Product
  Product2 : Product
  Sout : Display
      settings: Format=short_e
  Terminator3 : Terminator
  Trigonometric Function : Trigonometry  Operator=cos
  "Vllrms " : Display
  pf : Display
  wires:
  Gain8/1 -> Product1/1, "Vllrms "/1
  Gain9/1 -> "Ilinerms "/1, Product1/2
  Ia/1 -> Fourier1/1
  Fourier1/1 -> Gain9/1
  Vab/1 -> Fourier/1
  Fourier/1 -> Gain8/1
  Product1/1 -> Gain/1
  Gain/1 -> Product2/1, Sout/1
  Fourier1/2 -> Gain1/1, Display8/1
  Trigonometric Function/1 -> Product2/2, pf/1
  Gain1/1 -> Trigonometric Function/1
  Product2/1 -> Pout/1
  Fourier/2 -> Terminator3/1

== system topology2_module/Subsystem5 ==
  Vab : Inport
  Ia : Inport  Port=2
  Display8 : Display
  Fourier : powerlib_meascontrol/Measurements/Fourier  Freq=fout  n=1  InInit=[0, 0]  Ts=Ts
  Fourier1 : powerlib_meascontrol/Measurements/Fourier  Freq=fout  n=1  InInit=[0, 0]  Ts=Ts
  Gain : Gain  Gain=sqrt(3)
  Gain1 : Gain  Gain=pi/180
  Gain8 : Gain  Gain=1/sqrt(2)
  Gain9 : Gain  Gain=1/sqrt(2)
  "Ilinerms " : Display
  Pout : Display
  Product1 : Product
  Product2 : Product
  Sout : Display
      settings: Format=short_e
  Terminator3 : Terminator
  Trigonometric Function : Trigonometry  Operator=cos
  "Vllrms " : Display
  pf : Display
  wires:
  Gain8/1 -> Product1/1, "Vllrms "/1
  Gain9/1 -> "Ilinerms "/1, Product1/2
  Ia/1 -> Fourier1/1
  Fourier1/1 -> Gain9/1
  Vab/1 -> Fourier/1
  Fourier/1 -> Gain8/1
  Product1/1 -> Gain/1
  Gain/1 -> Product2/1, Sout/1
  Fourier1/2 -> Gain1/1, Display8/1
  Trigonometric Function/1 -> Product2/2, pf/1
  Gain1/1 -> Trigonometric Function/1
  Product2/1 -> Pout/1
  Fourier/2 -> Terminator3/1

== system topology2_module/Subsystem6 ==
  Vab : Inport
  Ia : Inport  Port=2
  Display8 : Display
  Fourier : powerlib_meascontrol/Measurements/Fourier  Freq=fout  n=1  InInit=[0, 0]  Ts=Ts
  Fourier1 : powerlib_meascontrol/Measurements/Fourier  Freq=fout  n=1  InInit=[0, 0]  Ts=Ts
  Gain : Gain  Gain=sqrt(3)
  Gain1 : Gain  Gain=pi/180
  Gain8 : Gain  Gain=1/sqrt(2)
  Gain9 : Gain  Gain=1/sqrt(2)
  "Ilinerms " : Display
  Pout : Display
  Product1 : Product
  Product2 : Product
  Sout : Display
      settings: Format=short_e
  Terminator3 : Terminator
  Trigonometric Function : Trigonometry  Operator=cos
  "Vllrms " : Display
  pf : Display
  wires:
  Gain8/1 -> Product1/1, "Vllrms "/1
  Gain9/1 -> "Ilinerms "/1, Product1/2
  Ia/1 -> Fourier1/1
  Fourier1/1 -> Gain9/1
  Vab/1 -> Fourier/1
  Fourier/1 -> Gain8/1
  Product1/1 -> Gain/1
  Gain/1 -> Product2/1, Sout/1
  Fourier1/2 -> Gain1/1, Display8/1
  Trigonometric Function/1 -> Product2/2, pf/1
  Gain1/1 -> Trigonometric Function/1
  Product2/1 -> Pout/1
  Fourier/2 -> Terminator3/1

== system topology2_module/Subsystem7 ==
  Vab : Inport
  Ia : Inport  Port=2
  Display8 : Display
  Fourier : powerlib_meascontrol/Measurements/Fourier  Freq=fout  n=1  InInit=[0, 0]  Ts=Ts
  Fourier1 : powerlib_meascontrol/Measurements/Fourier  Freq=fout  n=1  InInit=[0, 0]  Ts=Ts
  Gain : Gain  Gain=sqrt(3)
  Gain1 : Gain  Gain=pi/180
  Gain8 : Gain  Gain=1/sqrt(2)
  Gain9 : Gain  Gain=1/sqrt(2)
  "Ilinerms " : Display
  Pout : Display
  Product1 : Product
  Product2 : Product
  Sout : Display
      settings: Format=short_e
  Terminator3 : Terminator
  Trigonometric Function : Trigonometry  Operator=cos
  "Vllrms " : Display
  pf : Display
  wires:
  Gain8/1 -> Product1/1, "Vllrms "/1
  Gain9/1 -> "Ilinerms "/1, Product1/2
  Ia/1 -> Fourier1/1
  Fourier1/1 -> Gain9/1
  Vab/1 -> Fourier/1
  Fourier/1 -> Gain8/1
  Product1/1 -> Gain/1
  Gain/1 -> Product2/1, Sout/1
  Fourier1/2 -> Gain1/1, Display8/1
  Trigonometric Function/1 -> Product2/2, pf/1
  Gain1/1 -> Trigonometric Function/1
  Product2/1 -> Pout/1
  Fourier/2 -> Terminator3/1
